simulink model "VerificaAssegnamentoAutoval_11032026"  (R2025b)
settings: Solver=VariableStepAuto  StartTime=0.0  StopTime=15.0  RelTol=1e-3
values from neighbouring files (symbols this model uses):
  A = double(subs(A_sym, x, x_star))    [SvolgimentoEsame_11032026.m]
  B = double(subs(B_sym, x, x_star))    [SvolgimentoEsame_11032026.m]
  C = eye(4)    [SvolgimentoEsame_11032026.m]
  D = zeros(4, 2)    [SvolgimentoEsame_11032026.m]
  K = place(A, B, p)    [SvolgimentoEsame_11032026.m]
  N = -inv(C_N * (A_cl \ B))    [SvolgimentoEsame_11032026.m]
  x_0 = [q1_0 ... (first row only)    [SvolgimentoEsame_11032026.m]
  x_ref = [q1_ref ... (first row only)    [SvolgimentoEsame_11032026.m]
settings Model: Creator=salvo  LastModifiedBy=salvo

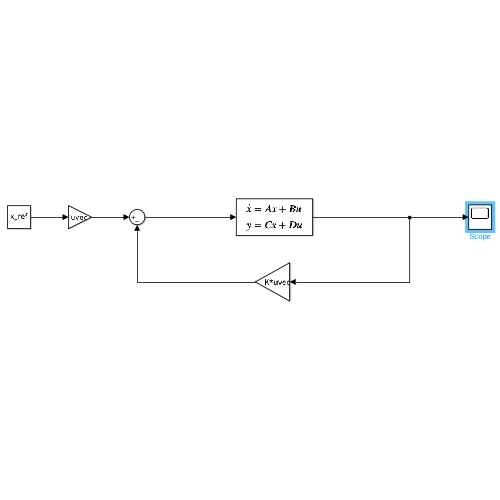
[thumbnail: Simulink's stored preview of the top-level diagram]
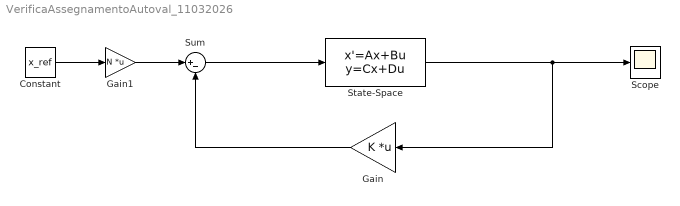
== system VerificaAssegnamentoAutoval_11032026 ==
  Constant : Constant  Value=x_ref
  Gain : Gain  Gain=K  Multiplication=Matrix(K*u) (u vector)
  Gain1 : Gain  Gain=N  Multiplication=Matrix(K*u) (u vector)
  Scope : Scope
      settings: ActiveDisplayYMinimum=-7.6071319604566918  ActiveDisplayYMaximum=10.921087745684723
  State-Space : StateSpace  A=A  B=B  C=C  D=D  InitialCondition=x_0
  Sum : Sum  Inputs=|+-
  wires:
  Constant/1 -> Gain1/1
  Gain/1 -> Sum/2
  Gain1/1 -> Sum/1
  State-Space/1 -> Gain/1, Scope/1
  Sum/1 -> State-Space/1
